simulink model "single_flight"  (R2019b)
settings: Solver=FixedStepAuto  StartTime=0.0  StopTime=100.0  FixedStep=0.01  RelTol=1e-3
values from neighbouring files (symbols this model uses):
  centerHeigt = 1    [calculator.m]    (also in flight_details.m; landing_dimensions.m; required_speed.m = 0; single_fly.m)
  speed = StartSpeeds(n)    [calculator.m]    (also in flight_details.m = 11.1111111111; landing_dimensions.m; required_speed.m = sqrt(speed^2 + 2*G*rampHeight); single_fly.m = 22.2222222222)
libraries: simulink x1
settings Model: Creator=Zver  LastModifiedBy=Zver

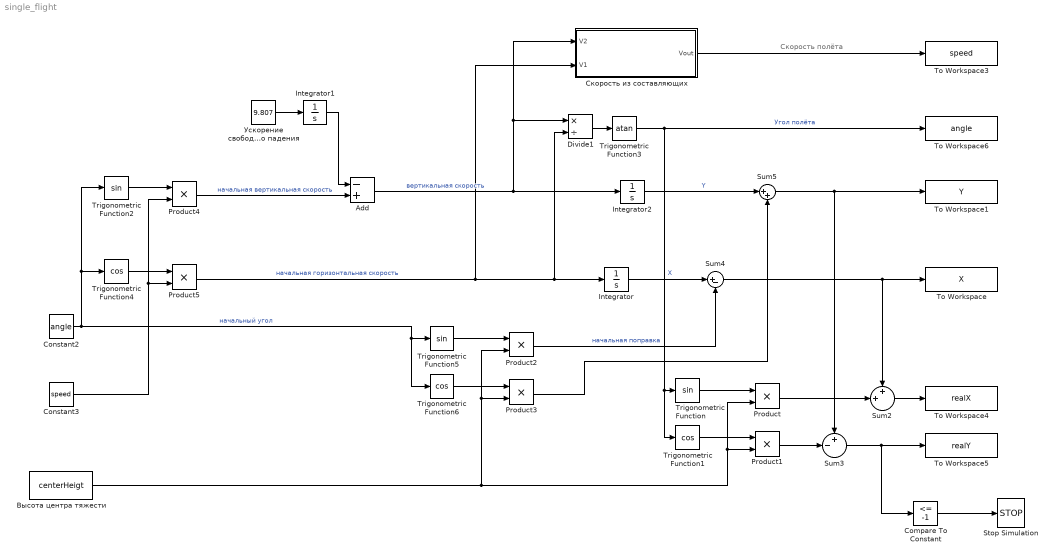
== system single_flight ==
  note: Скорость полёта
  Add : Sum  Inputs=-+
  Compare To Constant : simulink/Logic and Bit Operations/Compare To Constant  relop=<=  const=-1  OutDataTypeStr=boolean
  Constant2 : Constant  Value=angle
  Constant3 : Constant  Value=speed
  Divide1 : Product  Inputs=*/
  Integrator : Integrator
  Integrator1 : Integrator
  Integrator2 : Integrator
  Product{,1..5} (6 alike) : Product
  Stop Simulation : Stop
  Sum2 : Sum  Inputs=++|
  Sum3 : Sum  Inputs=+-|
  Sum4 : Sum  Inputs=|+-
  Sum5 : Sum  Inputs=|++
  To Workspace : ToWorkspace  VariableName=X  SaveFormat=Timeseries  SampleTime=-1
  To Workspace1 : ToWorkspace  VariableName=Y  SaveFormat=Timeseries  SampleTime=-1
  To Workspace3 : ToWorkspace  VariableName=speed  SaveFormat=Timeseries  SampleTime=-1
  To Workspace4 : ToWorkspace  VariableName=realX  SaveFormat=Timeseries  SampleTime=-1
  To Workspace5 : ToWorkspace  VariableName=realY  SaveFormat=Timeseries  SampleTime=-1
  To Workspace6 : ToWorkspace  VariableName=angle  SaveFormat=Timeseries  SampleTime=-1
  Trigonometric Function : Trigonometry
  Trigonometric Function1 : Trigonometry  Operator=cos
  Trigonometric Function2 : Trigonometry
  Trigonometric Function3 : Trigonometry  Operator=atan
  Trigonometric Function4 : Trigonometry  Operator=cos
  Trigonometric Function5 : Trigonometry
  Trigonometric Function6 : Trigonometry  Operator=cos
  "Высота центра тяжести " : Constant  Value=centerHeigt
  Скорость из составляющих : Subsystem
  Ускорение свободного падения : Constant  Value=9.807
  wires:
  Product5/1 -> Скорость из составляющих/2(V1), Divide1/2, Integrator/1  "начальная горизонтальная скорость"
  Ускорение свободного падения/1 -> Integrator1/1
  Product4/1 -> Add/2  "начальная вертикальная скорость"
  Integrator1/1 -> Add/1
  Add/1 -> Скорость из составляющих/1(V2), Divide1/1, Integrator2/1  "вертикальная скорость"
  Compare To Constant/1 -> Stop Simulation/1
  Divide1/1 -> Trigonometric Function3/1
  Trigonometric Function3/1 -> To Workspace6/1, Trigonometric Function1/1, Trigonometric Function/1  "Угол полёта"
  Trigonometric Function1/1 -> Product1/1
  Trigonometric Function/1 -> Product/1
  Product/1 -> Sum2/2
  Sum2/1 -> To Workspace4/1
  Product1/1 -> Sum3/2
  Sum3/1 -> Compare To Constant/1, To Workspace5/1
  "Высота центра тяжести "/1 -> Product3/2, Product2/2, Product/2, Product1/2
  Trigonometric Function6/1 -> Product3/1
  Trigonometric Function5/1 -> Product2/1
  Constant2/1 -> Trigonometric Function2/1, Trigonometric Function4/1, Trigonometric Function6/1, Trigonometric Function5/1  "начальный угол"
  Integrator/1 -> Sum4/1  "X"
  Product2/1 -> Sum4/2  "начальная поправка"
  Sum4/1 -> Sum2/1, To Workspace/1
  Integrator2/1 -> Sum5/1  "Y"
  Sum5/1 -> Sum3/1, To Workspace1/1
  Product3/1 -> Sum5/2
  Скорость из составляющих/1(Vout) -> To Workspace3/1
  Trigonometric Function2/1 -> Product4/1
  Trigonometric Function4/1 -> Product5/1
  Constant3/1 -> Product4/2, Product5/2

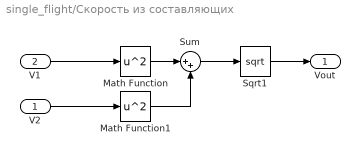
== system single_flight/Скорость из составляющих ==
  V2 : Inport
  V1 : Inport  Port=2
  Math Function : Math  Operator=square  SignedPower=off  SaturateOnIntegerOverflow=on
  Math Function1 : Math  Operator=square  SignedPower=off  SaturateOnIntegerOverflow=on
  Sqrt1 : Sqrt  SaturateOnIntegerOverflow=on
  Sum : Sum  Inputs=|++
  Vout : Outport
  wires:
  Math Function1/1 -> Sum/2
  Math Function/1 -> Sum/1
  Sum/1 -> Sqrt1/1
  Sqrt1/1 -> Vout/1
  V1/1 -> Math Function/1
  V2/1 -> Math Function1/1
